simulink subsystem "YawStateObserver_SubSystem"  (R2020b)
settings: Solver=VariableStepAuto  StartTime=0.0  StopTime=10.0  RelTol=1e-3
undefined symbols (not defined in the file): gbox, Hw, sens, Ts, wheel
settings Model: Creator=umberto  LastModifiedBy=Musta

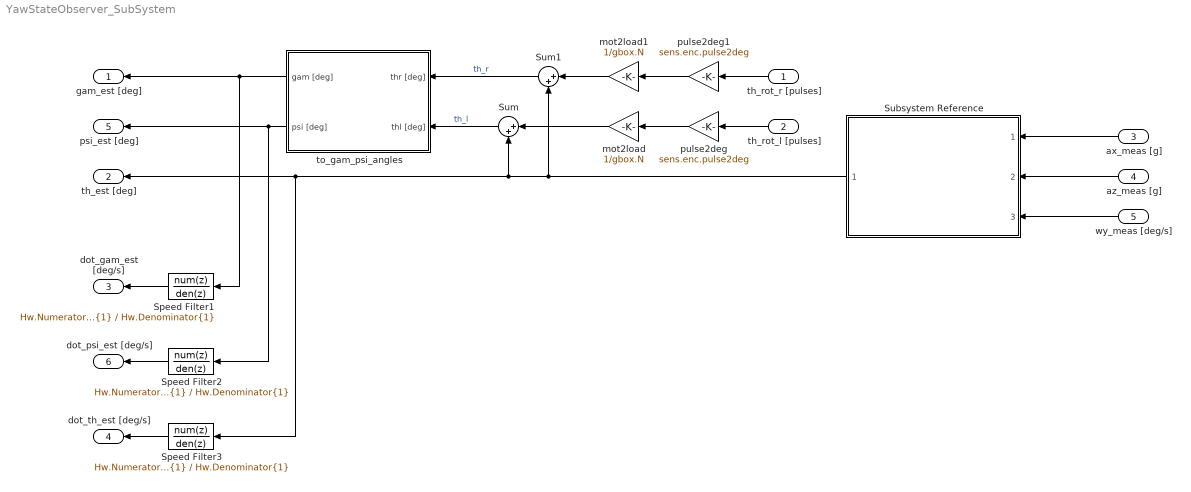
== system YawStateObserver_SubSystem ==
  th_rot_r [pulses] : Inport
  th_rot_l [pulses] : Inport  Port=2
  ax_meas [g] : Inport  Port=3
  az_meas [g] : Inport  Port=4
  wy_meas [deg/s] : Inport  Port=5
  Speed Filter1 : DiscreteTransferFcn  Numerator=Hw.Numerator{1}  Denominator=Hw.Denominator{1}  SampleTime=Ts
  Speed Filter2 : DiscreteTransferFcn  Numerator=Hw.Numerator{1}  Denominator=Hw.Denominator{1}  SampleTime=Ts
  Speed Filter3 : DiscreteTransferFcn  Numerator=Hw.Numerator{1}  Denominator=Hw.Denominator{1}  SampleTime=Ts
  Subsystem Reference : Subsystem  ReferencedSubsystem=CF1_SubSystem
  Sum : Sum  Inputs=|++
  Sum1 : Sum  Inputs=|++
  mot2load : Gain  Gain=1/gbox.N
  mot2load1 : Gain  Gain=1/gbox.N
  pulse2deg : Gain  Gain=sens.enc.pulse2deg
  pulse2deg1 : Gain  Gain=sens.enc.pulse2deg
  to_gam_psi_angles : Subsystem
  gam_est [deg] : Outport
  th_est [deg] : Outport  Port=2
  dot_gam_est [deg/s] : Outport  Port=3
  dot_th_est [deg/s] : Outport  Port=4
  psi_est [deg] : Outport  Port=5
  dot_psi_est [deg/s] : Outport  Port=6
  wires:
  ax_meas [g]/1 -> Subsystem Reference/1
  az_meas [g]/1 -> Subsystem Reference/2
  wy_meas [deg/s]/1 -> Subsystem Reference/3
  th_rot_l [pulses]/1 -> pulse2deg/1
  pulse2deg/1 -> mot2load/1
  mot2load/1 -> Sum/1
  Subsystem Reference/1 -> Sum1/2, Sum/2, Speed Filter3/1, th_est [deg]/1
  Speed Filter1/1 -> dot_gam_est [deg/s]/1
  Speed Filter2/1 -> dot_psi_est [deg/s]/1
  th_rot_r [pulses]/1 -> pulse2deg1/1
  mot2load1/1 -> Sum1/1
  pulse2deg1/1 -> mot2load1/1
  Speed Filter3/1 -> dot_th_est [deg/s]/1
  to_gam_psi_angles/1(gam [deg]) -> gam_est [deg]/1, Speed Filter1/1
  to_gam_psi_angles/2(psi [deg]) -> psi_est [deg]/1, Speed Filter2/1
  Sum/1 -> to_gam_psi_angles/2(thl [deg])  "th_l"
  Sum1/1 -> to_gam_psi_angles/1(thr [deg])  "th_r"

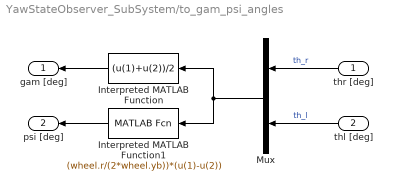
== system YawStateObserver_SubSystem/to_gam_psi_angles ==
  thr [deg] : Inport
  thl [deg] : Inport  Port=2
  Interpreted MATLAB Function : MATLABFcn  MATLABFcn=(u(1)+u(2))/2
  Interpreted MATLAB Function1 : MATLABFcn  MATLABFcn=(wheel.r/(2*wheel.yb))*(u(1)-u(2))
  Mux : Mux  Inputs=2
  gam [deg] : Outport
  psi [deg] : Outport  Port=2
  wires:
  Mux/1 -> Interpreted MATLAB Function/1, Interpreted MATLAB Function1/1
  Interpreted MATLAB Function1/1 -> psi [deg]/1
  Interpreted MATLAB Function/1 -> gam [deg]/1
  thl [deg]/1 -> Mux/2  "th_l"
  thr [deg]/1 -> Mux/1  "th_r"
